simulink model "non_linear_model"  (Simulink 5.0)
settings: Solver=ode45  StartTime=0.0  StopTime=0.01  FixedStep=0.000001  RelTol=1e-1
libraries: simulink x3
settings Model: LastModifiedBy=Admin  OptimizeBlockIOStorage=off  RTWOptions="-aEnforceIntegerDowncast=1 -aExtMode=0 -aExtModeTesting=0 -aFoldNonRolledExpr=1 -aForceParamTrailComments=0 -aGenerateComments=1 -aGenerateReport=0 -aIgnoreCustomStorageClasses=1 -aIncDataTypeInIds=0 -aIncHierarchyInIds=0 -aInlineInvariantSignals=1 -aInlineParameters=0 -aInlinedPrmAccess=\"Literals\" -aLocalBlockOutputs=1 -aLogVarNameModifier=\"rt_\" -aMaxRTWIdLen=31 -aPrefixModelToSubsysFcnNames=1 -aRTWVerbose=1 -aRollThreshold=5 -aShowEliminatedStatements=0"

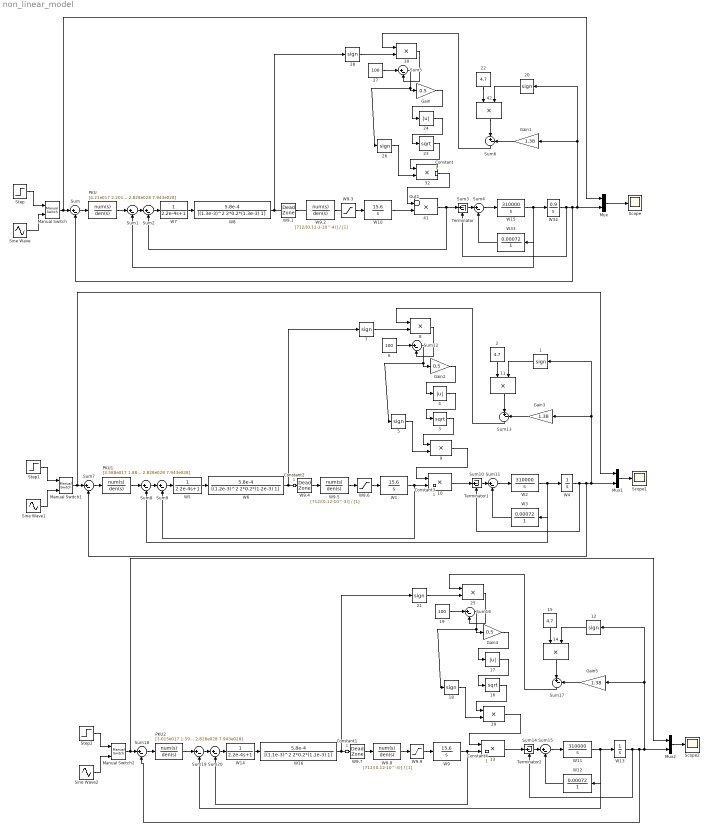
== system non_linear_model ==
  1 : Signum  Orientation=left
  {8..10,13,25,29..30,32,41} (9 alike) : Product  SaturateOnIntegerOverflow=on
  11 : Product  Orientation=down  SaturateOnIntegerOverflow=on
  12 : Signum  Orientation=left
  14 : Product  Orientation=down  SaturateOnIntegerOverflow=on
  15 : Constant  Orientation=down  Value=4.7
  16 : Math  Operator=sqrt
  17 : Abs  SaturateOnIntegerOverflow=on
  {5,7,18,21,26,28} (6 alike) : Signum
  19 : Constant  Value=100
  2 : Constant  Orientation=down  Value=4.7
  20 : Signum  Orientation=left
  22 : Constant  Orientation=down  Value=4.7
  23 : Math  Operator=sqrt
  24 : Abs  SaturateOnIntegerOverflow=on
  27 : Constant  Value=100
  3 : Math  Operator=sqrt
  4 : Abs  SaturateOnIntegerOverflow=on
  42 : Product  Orientation=down  SaturateOnIntegerOverflow=on
  6 : Constant  Value=100
  Constant{,1..4} (5 alike) : Constant
  Gain : Gain  Gain=0.5  SaturateOnIntegerOverflow=on
  Gain1 : Gain  Orientation=left  Gain=1.38  SaturateOnIntegerOverflow=on
  Gain2 : Gain  Gain=0.5  SaturateOnIntegerOverflow=on
  Gain3 : Gain  Orientation=left  Gain=1.38  SaturateOnIntegerOverflow=on
  Gain4 : Gain  Gain=0.5  SaturateOnIntegerOverflow=on
  Gain5 : Gain  Orientation=left  Gain=1.38  SaturateOnIntegerOverflow=on
  Manual Switch : simulink/Signal Routing/Manual Switch  sw=0  action=0
  Manual Switch1 : simulink/Signal Routing/Manual Switch  sw=1  action=0
  Manual Switch2 : simulink/Signal Routing/Manual Switch  sw=1  action=0
  Mux : Mux  Inputs=2
  Mux1 : Mux  Inputs=2
  Mux2 : Mux  Inputs=2
  PKU : TransferFcn  Numerator="[4.21e017 2.201e021 1.745e024 2.167e027 8.056e029  4.28e032 5.268e034 9.532e032]"  Denominator=[1 1.539e006 8.565e011 2.152e017 2.439e022 1.001e027 2.828e028 7.943e028]
  PKU1 : TransferFcn  Numerator="[3.588e017 1.884e021 1.569e024  2.046e027  7.764e029 4.259e032 5.268e034 9.532e032]"  Denominator=[1 1.539e006 8.565e011 2.152e017 2.439e022 1.001e027 2.828e028 7.943e028]
  PKU2 : TransferFcn  Numerator=[3.015e017 1.592e021 1.403e024 1.934e027 7.482e029 4.237e032 5.268e034 9.532e032]  Denominator=[1 1.539e006 8.565e011 2.152e017 2.439e022 1.001e027 2.828e028 7.943e028]
  Scope : Scope
      settings: TimeRange=0.003  YMin=0  YMax=1.2
  Scope1 : Scope
      settings: TimeRange=0.01  YMin=1  YMax=1.03
  Scope2 : Scope
      settings: TimeRange=0.01  YMin=-1  YMax=1  SaveName=ScopeData2
  Sine Wave : Sin  Frequency=1500  SampleTime=0
  Sine Wave1 : Sin  Frequency=1200  SampleTime=0
  Sine Wave2 : Sin  Frequency=1200  SampleTime=0
  Step : Step  Time=0  SampleTime=0
  Step1 : Step  Time=0  SampleTime=0
  Step2 : Step  Time=0  SampleTime=0
  Sum{,1..5,7..12,14..16,18..20} (18 alike) : Sum  Inputs=|+-  SaturateOnIntegerOverflow=on
  Sum13 : Sum  Orientation=down  Inputs=|+-  SaturateOnIntegerOverflow=on
  Sum17 : Sum  Orientation=down  Inputs=|+-  SaturateOnIntegerOverflow=on
  Sum6 : Sum  Orientation=down  Inputs=|+-  SaturateOnIntegerOverflow=on
  Terminator : Terminator
  Terminator1 : Terminator
  Terminator2 : Terminator
  W1 : TransferFcn  Numerator=[15.6]  Denominator=[1 0]
  W10 : TransferFcn  Numerator=[15.6]  Denominator=[1 0]
  W11 : TransferFcn  Numerator=[310000]  Denominator=[1 0]
  W12 : TransferFcn  Orientation=left  Numerator=[0.00072]  Denominator=[1]
  W13 : TransferFcn  Denominator=[1 0]
  W14 : TransferFcn  Denominator=[2.2e-4 1]
  W15 : TransferFcn  Numerator=[310000]  Denominator=[1 0]
  W16 : TransferFcn  Numerator=[5.8e-4]  Denominator=[(1.1e-3)^2 2*0.2*(1.1e-3) 1]
  W2 : TransferFcn  Numerator=[310000]  Denominator=[1 0]
  W3 : TransferFcn  Orientation=left  Numerator=[0.00072]  Denominator=[1]
  W33 : TransferFcn  Orientation=left  Numerator=[0.00072]  Denominator=[1]
  W34 : TransferFcn  Numerator=[0.9]  Denominator=[1 0]
  W4 : TransferFcn  Denominator=[1 0]
  W5 : TransferFcn  Denominator=[2.2e-4 1]
  W6 : TransferFcn  Numerator=[5.8e-4]  Denominator=[(1.2e-3)^2 2*0.2*(1.2e-3) 1]
  W7 : TransferFcn  Denominator=[2.2e-4 1]
  W8 : TransferFcn  Numerator=[5.8e-4]  Denominator=[(1.3e-3)^2 2*0.2*(1.3e-3) 1]
  W9 : TransferFcn  Numerator=[15.6]  Denominator=[1 0]
  W9.1 : DeadZone  LowerValue=-2-10^-3  UpperValue=2-10^-3  SaturateOnIntegerOverflow=on
  W9.2 : TransferFcn  Numerator=[712/(0.12-2-10^-4)]  Denominator=[1]
  W9.3 : Saturate  UpperLimit=1190  LowerLimit=-1190
  W9.4 : DeadZone  LowerValue=-2*10^-3  UpperValue=2*10^-3  SaturateOnIntegerOverflow=on
  W9.5 : TransferFcn  Numerator=[712/(0.12-10^-3)]  Denominator=[1]
  W9.6 : Saturate  UpperLimit=1190  LowerLimit=-1190
  W9.7 : DeadZone  LowerValue=-2*10^-3  UpperValue=2*10^-3  SaturateOnIntegerOverflow=on
  W9.8 : TransferFcn  Numerator=[712/(0.12-10^-3)]  Denominator=[1]
  W9.9 : Saturate  UpperLimit=1190  LowerLimit=-1190
  Out1 : Outport
  wires:
  Sum2/1 -> W7/1
  W7/1 -> W8/1
  Sum3/1 -> Sum4/1
  Sum4/1 -> W15/1
  W15/1 -> Sum1/2, W34/1, W33/1
  Step/1 -> Manual Switch/1
  Sine Wave/1 -> Manual Switch/2
  Mux/1 -> Scope/1
  Manual Switch/1 -> Mux/1, Sum/1
  Sum1/1 -> Sum2/1
  Sum/1 -> PKU/1
  W34/1 -> Sum3/2, Sum/2, Mux/2, Gain1/1, 20/1
  W33/1 -> Sum4/2
  PKU/1 -> Sum1/1
  23/1 -> 32/1
  24/1 -> 23/1
  Gain/1 -> 24/1
  26/1 -> 32/2
  Sum5/1 -> Gain/1, 26/1
  27/1 -> Sum5/1
  30/1 -> Sum5/2
  28/1 -> 30/2
  22/1 -> 42/1
  20/1 -> 42/2
  42/1 -> Sum6/1
  Gain1/1 -> Sum6/2
  Sum6/1 -> 30/1
  W8/1 -> 28/1, W10/1
  Sum9/1 -> W5/1
  W5/1 -> W6/1
  Sum10/1 -> Sum11/1
  Sum11/1 -> W2/1
  W2/1 -> Sum8/2, W4/1, W3/1
  Step1/1 -> Manual Switch1/1
  Sine Wave1/1 -> Manual Switch1/2
  Mux1/1 -> Scope1/1
  Manual Switch1/1 -> Mux1/1, Sum7/1
  Sum8/1 -> Sum9/1
  Sum7/1 -> PKU1/1
  W4/1 -> Sum10/2, Sum7/2, Mux1/2, Gain3/1, 1/1
  W3/1 -> Sum11/2
  PKU1/1 -> Sum8/1
  3/1 -> 9/1
  4/1 -> 3/1
  Gain2/1 -> 4/1
  5/1 -> 9/2
  Sum12/1 -> Gain2/1, 5/1
  6/1 -> Sum12/1
  8/1 -> Sum12/2
  7/1 -> 8/2
  2/1 -> 11/1
  1/1 -> 11/2
  11/1 -> Sum13/1
  Gain3/1 -> Sum13/2
  Sum13/1 -> 8/1
  9/1 -> 10/1
  W9.5/1 -> W9.6/1
  W6/1 -> W9.4/1, 7/1
  10/1 -> Terminator1/1
  W1/1 -> Sum9/2, Sum10/1
  W9.4/1 -> W1/1
  W9.6/1 -> 10/2
  Constant2/1 -> W9.5/1
  W9.1/1 -> W9.1/1
  W9.2/1 -> W9.2/1
  W9.3/1 -> W9.3/1
  Constant/1 -> 41/1
  W10/1 -> 41/2
  41/1 -> Sum3/1, Sum2/2
  32/1 -> Out1/1
  Sum20/1 -> W14/1
  W14/1 -> W16/1
  Sum14/1 -> Sum15/1
  Sum15/1 -> W11/1
  W11/1 -> Sum19/2, W13/1, W12/1
  Step2/1 -> Manual Switch2/1
  Sine Wave2/1 -> Manual Switch2/2
  Mux2/1 -> Scope2/1
  Manual Switch2/1 -> Mux2/1, Sum18/1
  Sum19/1 -> Sum20/1
  Sum18/1 -> PKU2/1
  W13/1 -> Sum14/2, Sum18/2, Mux2/2, Gain5/1, 12/1
  W12/1 -> Sum15/2
  PKU2/1 -> Sum19/1
  16/1 -> 29/1
  17/1 -> 16/1
  Gain4/1 -> 17/1
  18/1 -> 29/2
  Sum16/1 -> Gain4/1, 18/1
  19/1 -> Sum16/1
  25/1 -> Sum16/2
  21/1 -> 25/2
  15/1 -> 14/1
  12/1 -> 14/2
  14/1 -> Sum17/1
  Gain5/1 -> Sum17/2
  Sum17/1 -> 25/1
  29/1 -> 13/1
  W9.8/1 -> W9.9/1
  W16/1 -> W9.7/1, 21/1
  13/1 -> Terminator2/1
  W9/1 -> Sum20/2, Sum14/1
  W9.7/1 -> W9/1
  W9.9/1 -> 13/2
  Constant1/1 -> W9.8/1
